simulink model "model4_3_1"  (R2019b)
settings: Solver=VariableStepAuto  StartTime=0.0  StopTime=10.0  RelTol=1e-3
values from neighbouring files (symbols this model uses):
  a = A(n)    [lab4_3.m]
  f = F(n)    [lab4_3.m]    (also in lab4_4.m = (1/10)*fgr)
  w = W(n)    [lab4_3.m]
settings Model: Creator=marci  LastModifiedBy=marci

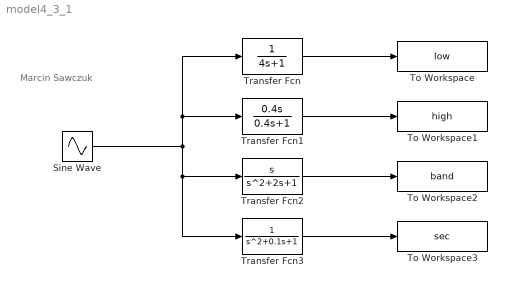
== system model4_3_1 ==
  note: Marcin Sawczuk
  Sine Wave : Sin  Amplitude=a  Frequency=w  Phase=f  SampleTime=0
  To Workspace : ToWorkspace  VariableName=low  SaveFormat=Timeseries  SampleTime=-1
  To Workspace1 : ToWorkspace  VariableName=high  SaveFormat=Timeseries  SampleTime=-1
  To Workspace2 : ToWorkspace  VariableName=band  SaveFormat=Timeseries  SampleTime=-1
  To Workspace3 : ToWorkspace  VariableName=sec  SaveFormat=Timeseries  SampleTime=-1
  Transfer Fcn : TransferFcn  Denominator=[4 1]
  Transfer Fcn1 : TransferFcn  Numerator=[0.4 0]  Denominator=[0.4 1]
  Transfer Fcn2 : TransferFcn  Numerator=[1 0]
  Transfer Fcn3 : TransferFcn  Denominator=[1 0.1 1]
  wires:
  Transfer Fcn/1 -> To Workspace/1
  Transfer Fcn1/1 -> To Workspace1/1
  Transfer Fcn2/1 -> To Workspace2/1
  Transfer Fcn3/1 -> To Workspace3/1
  Sine Wave/1 -> Transfer Fcn3/1, Transfer Fcn2/1, Transfer Fcn1/1, Transfer Fcn/1
